simulink model "ComissionamentoMesa_simul"  (R2024a)
settings: Solver=FixedStepDiscrete  StartTime=0.0  StopTime=50  FixedStep=50e-3  RelTol=1e-3
undefined symbols (not defined in the file): flap_front_left_down, flap_front_left_up, flap_front_right_down, flap_front_right_up, flap_rear_left_down, flap_rear_left_up, flap_rear_right_down, flap_rear_right_up, tstep
libraries: speedgoatlib_IO60X_IO69X x1, tramontina_database_curtis_mesalib x1
settings Model: Creator=matlab.cut  LastModifiedBy=matlab.cut

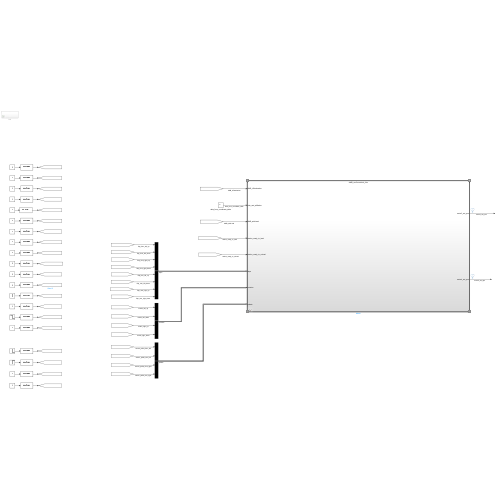
[thumbnail: Simulink's stored preview of the top-level diagram]
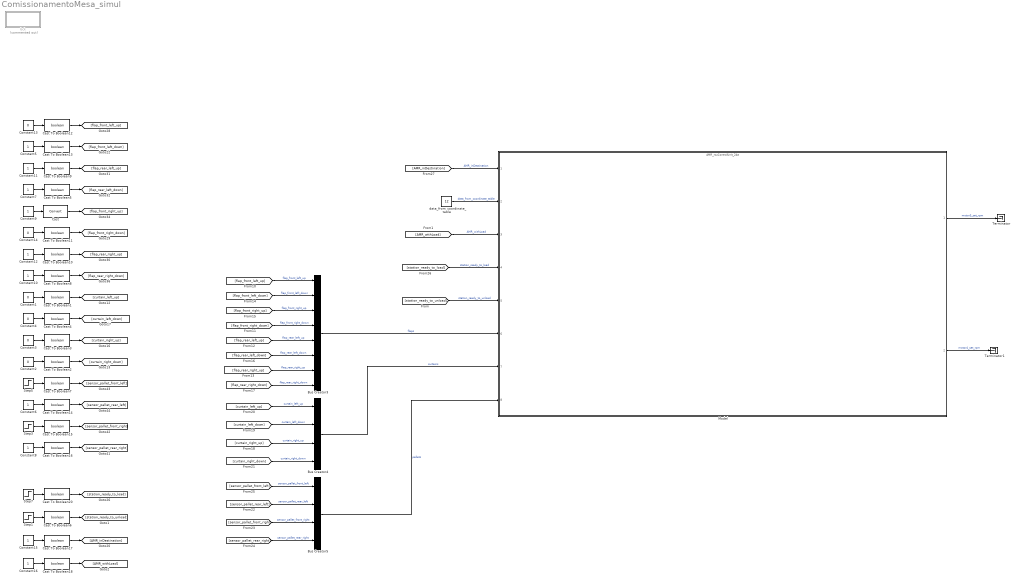
== system ComissionamentoMesa_simul ==
  Bus Creator3 : BusCreator  Inputs=flap_front_left_up,flap_front_left_down,flap_front_right_up,flap_front_right_down,flap_rear_left_up,flap_rear_left_down,flap_rear_right_up,flap_rear_right_down  OutDataTypeStr=Bus: IOs_flaps_bool
  Bus Creator4 : BusCreator  Inputs=4
  Bus Creator5 : BusCreator  Inputs=4
  Cast : DataTypeConversion  SaturateOnIntegerOverflow=off  RndMeth=Floor
  Cast To Boolean{1..18,20} (19 alike) : DataTypeConversion  OutDataTypeStr=boolean  SaturateOnIntegerOverflow=off  RndMeth=Floor
  Constant{1..4,13..14} (6 alike) : Constant  Value=0
  Constant{5..12,15..16} (10 alike) : Constant
  Model : ModelReference  ModelNameDialog=AMR_rcuControlUnit_24a.slx  SimulationMode=Normal  ModelReferenceVersion=1.13
  Step1 : Step  Time=40
  Step3 : Step  Time=35  Before=1  After=0  SampleTime=500e-3
  Step5 : Step  Time=35  Before=1  After=0  SampleTime=500e-3
  Step7 : Step  Time=30  Before=1  After=0
  Terminator : Terminator
  Terminator1 : Terminator
  bck : Subsystem  Commented=on
  data_from_coordinate_table : Constant  Value=12
  wires:
  Cast To Boolean7/1 -> [sensor_pallet_front_left]
  Step3/1 -> Cast To Boolean15/1
  Constant6/1 -> Cast To Boolean14/1
  Cast To Boolean15/1 -> [sensor_pallet_front_right]
  Cast To Boolean13/1 -> [flap_front_left_down]
  Constant5/1 -> Cast To Boolean13/1
  Constant13/1 -> Cast To Boolean12/1
  Constant10/1 -> Cast To Boolean8/1
  Cast To Boolean9/1 -> [flap_rear_left_up]
  Cast To Boolean11/1 -> [flap_front_right_down]
  Step5/1 -> Cast To Boolean7/1
  Cast To Boolean1/1 -> [curtain_left_up]
  Cast To Boolean14/1 -> [sensor_pallet_rear_left]
  Constant7/1 -> Cast To Boolean5/1
  Constant8/1 -> Cast To Boolean16/1
  Cast To Boolean10/1 -> [flap_rear_right_up]
  Cast To Boolean16/1 -> [sensor_pallet_rear_right]
  Constant11/1 -> Cast To Boolean9/1
  Constant14/1 -> Cast To Boolean11/1
  Constant2/1 -> Cast To Boolean2/1
  Cast To Boolean3/1 -> [curtain_right_up]
  Cast To Boolean4/1 -> [curtain_left_down]
  Constant3/1 -> Cast To Boolean3/1
  Cast To Boolean8/1 -> [flap_rear_right_down]
  Cast To Boolean2/1 -> [curtain_right_down]
  Constant1/1 -> Cast To Boolean1/1
  Cast To Boolean12/1 -> [flap_front_left_up]
  Cast To Boolean5/1 -> [flap_rear_left_down]
  Constant12/1 -> Cast To Boolean10/1
  Constant4/1 -> Cast To Boolean4/1
  [curtain_left_up] -> Bus Creator4/1  "curtain_left_up"
  [flap_front_left_down] -> Bus Creator3/2  "flap_front_left_down"
  [flap_rear_right_down] -> Bus Creator3/8  "flap_rear_right_down"
  [sensor_pallet_rear_right] -> Bus Creator5/4  "sensor_pallet_rear_right"
  [curtain_right_down] -> Bus Creator4/4  "curtain_right_down"
  [AMR_inDestination] -> Model/1  "AMR_inDestination"
  [flap_rear_right_up] -> Bus Creator3/7  "flap_rear_right_up"
  [flap_rear_left_down] -> Bus Creator3/6  "flap_rear_left_down"
  [sensor_pallet_front_right] -> Bus Creator5/3  "sensor_pallet_front_right"
  [flap_rear_left_up] -> Bus Creator3/5  "flap_rear_left_up"
  [flap_front_right_up] -> Bus Creator3/3  "flap_front_right_up"
  [flap_front_left_up] -> Bus Creator3/1  "flap_front_left_up"
  [sensor_pallet_rear_left] -> Bus Creator5/2  "sensor_pallet_rear_left"
  [sensor_pallet_front_left] -> Bus Creator5/1  "sensor_pallet_front_left"
  [curtain_right_up] -> Bus Creator4/3  "curtain_right_up"
  data_from_coordinate_table/1 -> Model/2  "data_from_coordinate_table"
  [flap_front_right_down] -> Bus Creator3/4  "flap_front_right_down"
  [curtain_left_down] -> Bus Creator4/2  "curtain_left_down"
  Constant15/1 -> Cast To Boolean17/1
  Cast To Boolean17/1 -> [AMR_inDestination]
  Cast To Boolean20/1 -> [station_ready_to_load]
  Step7/1 -> Cast To Boolean20/1
  Model/1 -> Terminator/1  "motor3_set_rpm"
  Model/2 -> Terminator1/1  "motor4_set_rpm"
  Cast/1 -> [flap_front_right_up]
  Constant9/1 -> Cast/1
  Cast To Boolean6/1 -> [station_ready_to_unload]
  Step1/1 -> Cast To Boolean6/1
  Cast To Boolean18/1 -> [AMR_withLoad]
  Constant16/1 -> Cast To Boolean18/1
  [AMR_withLoad] -> Model/3  "AMR_withLoad"
  [station_ready_to_load] -> Model/4  "station_ready_to_load"
  [station_ready_to_unload] -> Model/5  "station_ready_to_unload"
  Bus Creator3/1 -> Model/6  "flaps"
  Bus Creator4/1 -> Model/7  "curtains"
  Bus Creator5/1 -> Model/8  "pallets"

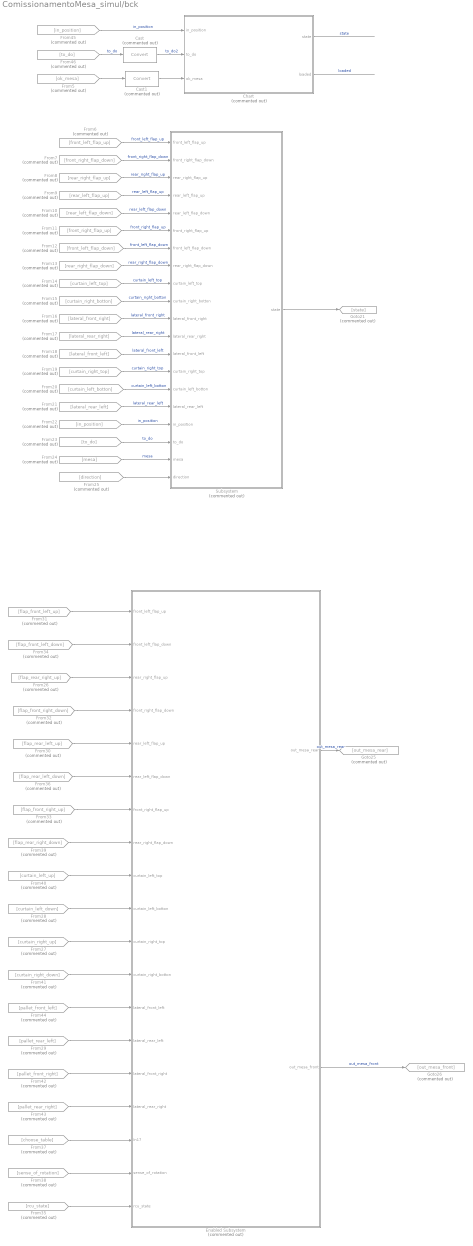
== system ComissionamentoMesa_simul/bck ==
  Cast : DataTypeConversion  Commented=on  SaturateOnIntegerOverflow=off  RndMeth=Floor
  Cast1 : DataTypeConversion  Commented=on  SaturateOnIntegerOverflow=off  RndMeth=Floor
  Chart : Stateflow chart  Commented=on  TreatAsAtomicUnit=on
  Enabled Subsystem : Subsystem  Commented=on  TreatAsAtomicUnit=on
  From10 : From  Commented=on  GotoTag=rear_left_flap_down
  From11 : From  Commented=on  GotoTag=front_right_flap_up
  From12 : From  Commented=on  GotoTag=front_left_flap_down
  From13 : From  Commented=on  GotoTag=rear_right_flap_down
  From14 : From  Commented=on  GotoTag=curtain_left_top
  From15 : From  Commented=on  GotoTag=curtain_right_botton
  From16 : From  Commented=on  GotoTag=lateral_front_right
  From17 : From  Commented=on  GotoTag=lateral_rear_right
  From18 : From  Commented=on  GotoTag=lateral_front_left
  From19 : From  Commented=on  GotoTag=curtain_right_top
  From20 : From  Commented=on  GotoTag=curtain_left_botton
  From21 : From  Commented=on  GotoTag=lateral_rear_left
  From22 : From  Commented=on  GotoTag=in_position
  From23 : From  Commented=on  GotoTag=to_do
  From24 : From  Commented=on  GotoTag=mesa
  From25 : From  Commented=on  GotoTag=direction
  From26 : From  Commented=on  GotoTag=flap_rear_right_up
  From27 : From  Commented=on  GotoTag=curtain_right_up
  From28 : From  Commented=on  GotoTag=curtain_left_down
  From29 : From  Commented=on  GotoTag=pallet_rear_left
  From30 : From  Commented=on  GotoTag=flap_rear_left_up
  From31 : From  Commented=on  GotoTag=flap_front_left_up
  From32 : From  Commented=on  GotoTag=flap_front_right_down
  From33 : From  Commented=on  GotoTag=flap_front_right_up
  From34 : From  Commented=on  GotoTag=flap_front_left_down
  From35 : From  Commented=on  GotoTag=rcu_state
  From36 : From  Commented=on  GotoTag=flap_rear_left_down
  From37 : From  Commented=on  GotoTag=choose_table
  From38 : From  Commented=on  GotoTag=sense_of_rotation
  From39 : From  Commented=on  GotoTag=flap_rear_right_down
  From40 : From  Commented=on  GotoTag=curtain_left_up
  From41 : From  Commented=on  GotoTag=curtain_right_down
  From42 : From  Commented=on  GotoTag=pallet_front_right
  From43 : From  Commented=on  GotoTag=pallet_rear_right
  From44 : From  Commented=on  GotoTag=pallet_front_left
  From45 : From  Commented=on  GotoTag=in_position
  From46 : From  Commented=on  GotoTag=to_do
  From5 : From  Commented=on  GotoTag=ok_mesa
  From6 : From  Commented=on  GotoTag=front_left_flap_up
  From7 : From  Commented=on  GotoTag=front_right_flap_down
  From8 : From  Commented=on  GotoTag=rear_right_flap_up
  From9 : From  Commented=on  GotoTag=rear_left_flap_up
  Goto21 : Goto  Commented=on  GotoTag=state
  Goto25 : Goto  Commented=on  GotoTag=out_mesa_rear
  Goto26 : Goto  Commented=on  GotoTag=out_mesa_front
  Subsystem : Subsystem  Commented=on
  wires:
  Chart/2(loaded) -> ?  "loaded"
  From31/1 -> Enabled Subsystem/1(front_left_flap_up)
  From27/1 -> Enabled Subsystem/11(curtain_right_top)
  From29/1 -> Enabled Subsystem/14(lateral_rear_left)
  From44/1 -> Enabled Subsystem/13(lateral_front_left)
  Enabled Subsystem/1(out_mesa_rear) -> Goto25/1  "out_mesa_rear"
  From30/1 -> Enabled Subsystem/5(rear_left_flap_up)
  From38/1 -> Enabled Subsystem/18(sense_of_rotation)
  From45/1 -> Chart/1(in_position)  "in_position"
  From6/1 -> Subsystem/1(front_left_flap_up)  "front_left_flap_up"
  Subsystem/1(state) -> Goto21/1
  From5/1 -> Cast1/1
  From43/1 -> Enabled Subsystem/16(lateral_rear_right)
  From32/1 -> Enabled Subsystem/4(front_right_flap_down)
  From13/1 -> Subsystem/8(rear_right_flap_down)  "rear_right_flap_down"
  From41/1 -> Enabled Subsystem/12(curtain_right_botton)
  From26/1 -> Enabled Subsystem/3(rear_right_flap_up)
  From34/1 -> Enabled Subsystem/2(front_left_flap_down)
  From20/1 -> Subsystem/15(curtain_left_botton)  "curtain_left_botton"
  From39/1 -> Enabled Subsystem/8(rear_right_flap_down)
  From37/1 -> Enabled Subsystem/17(In17)
  From24/1 -> Subsystem/19(mesa)  "mesa"
  From16/1 -> Subsystem/11(lateral_front_right)  "lateral_front_right"
  From22/1 -> Subsystem/17(in_position)  "in_position"
  From35/1 -> Enabled Subsystem/19(rcu_state)
  From42/1 -> Enabled Subsystem/15(lateral_front_right)
  From17/1 -> Subsystem/12(lateral_rear_right)  "lateral_rear_right"
  From21/1 -> Subsystem/16(lateral_rear_left)  "lateral_rear_left"
  From40/1 -> Enabled Subsystem/9(curtain_left_top)
  From14/1 -> Subsystem/9(curtain_left_top)  "curtain_left_top"
  Chart/1(state) -> ?  "state"
  From8/1 -> Subsystem/3(rear_right_flap_up)  "rear_right_flap_up"
  From18/1 -> Subsystem/13(lateral_front_left)  "lateral_front_left"
  From19/1 -> Subsystem/14(curtain_right_top)  "curtain_right_top"
  From10/1 -> Subsystem/5(rear_left_flap_down)  "rear_left_flap_down"
  From25/1 -> Subsystem/20(direction)
  From7/1 -> Subsystem/2(front_right_flap_down)  "front_right_flap_down"
  From46/1 -> Cast/1  "to_do"
  From9/1 -> Subsystem/4(rear_left_flap_up)  "rear_left_flap_up"
  Cast1/1 -> Chart/3(ok_mesa)
  From12/1 -> Subsystem/7(front_left_flap_down)  "front_left_flap_down"
  From28/1 -> Enabled Subsystem/10(curtain_left_botton)
  From11/1 -> Subsystem/6(front_right_flap_up)  "front_right_flap_up"
  Cast/1 -> Chart/2(to_do)  "to_do2"
  From15/1 -> Subsystem/10(curtain_right_botton)  "curtain_right_botton"
  From33/1 -> Enabled Subsystem/7(front_right_flap_up)
  From36/1 -> Enabled Subsystem/6(rear_left_flap_down)
  Enabled Subsystem/2(out_mesa_front) -> Goto26/1  "out_mesa_front"
  From23/1 -> Subsystem/18(to_do)  "to_do"

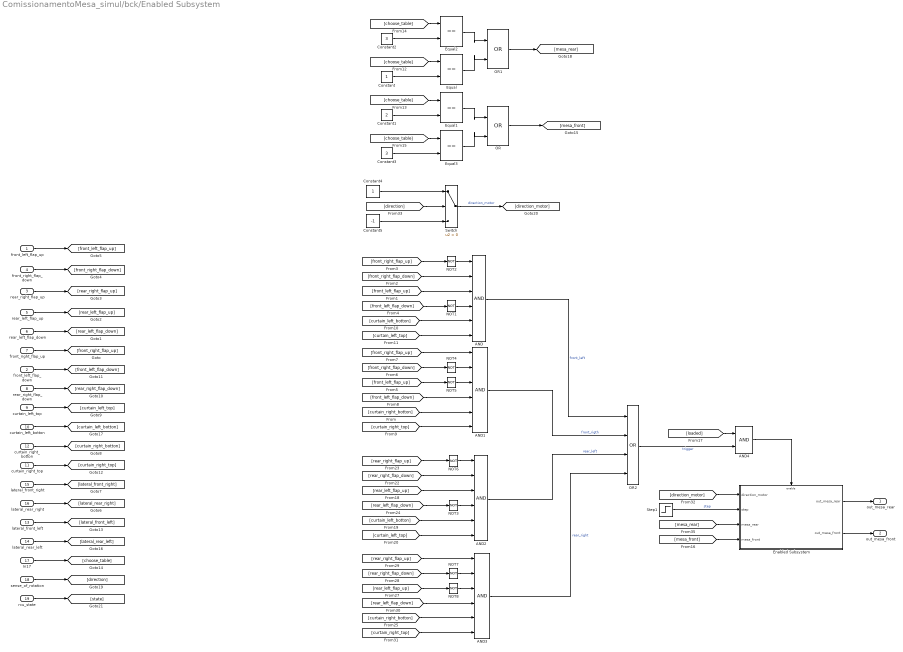
== system ComissionamentoMesa_simul/bck/Enabled Subsystem ==
  front_left_flap_up : Inport
  front_left_flap_down : Inport  Port=2
  rear_right_flap_up : Inport  Port=3
  front_right_flap_down : Inport  Port=4
  rear_left_flap_up : Inport  Port=5
  rear_left_flap_down : Inport  Port=6
  front_right_flap_up : Inport  Port=7
  rear_right_flap_down : Inport  Port=8
  curtain_left_top : Inport  Port=9
  curtain_left_botton : Inport  Port=10
  curtain_right_top : Inport  Port=11
  curtain_right_botton : Inport  Port=12
  lateral_front_left : Inport  Port=13
  lateral_rear_left : Inport  Port=14
  lateral_front_right : Inport  Port=15
  lateral_rear_right : Inport  Port=16
  In17 : Inport  Port=17
  sense_of_rotation : Inport  Port=18
  rcu_state : Inport  Port=19
  AND{,1..3} (4 alike) : Logic  Inputs=6  AllPortsSameDT=off  OutDataTypeStr=boolean
  AND4 : Logic  AllPortsSameDT=off  OutDataTypeStr=boolean
  Constant : Constant
  Constant1 : Constant  Value=2
  Constant2 : Constant  Value=3
  Constant3 : Constant  Value=3
  Constant4 : Constant
  Constant5 : Constant  Value=-1
  Enabled Subsystem : Subsystem  TreatAsAtomicUnit=on
  Equal{,1..3} (4 alike) : RelationalOperator  Operator===  OutDataTypeStr=boolean  RndMeth=Simplest  InputSameDT=off
  NOT{1..8} (8 alike) : Logic  Operator=NOT  IconShape=distinctive  AllPortsSameDT=off  OutDataTypeStr=boolean
  OR : Logic  Operator=OR  IconShape=distinctive  AllPortsSameDT=off  OutDataTypeStr=boolean
  OR1 : Logic  Operator=OR  IconShape=distinctive  AllPortsSameDT=off  OutDataTypeStr=boolean
  OR2 : Logic  Operator=OR  Inputs=4  AllPortsSameDT=off  OutDataTypeStr=boolean
  Step1 : Step  Time=20
  Switch : Switch  Criteria=u2 > Threshold  SaturateOnIntegerOverflow=off  InputSameDT=off
  out_mesa_rear : Outport
  out_mesa_front : Outport  Port=2
  wires:
  NOT2/1 -> AND/1
  [front_left_flap_up] -> AND/3
  NOT1/1 -> AND/4
  [front_left_flap_down] -> NOT1/1
  [front_right_flap_down] -> AND/2
  [front_right_flap_up] -> NOT2/1
  front_right_flap_down/1 -> [front_right_flap_down]
  front_left_flap_up/1 -> [front_left_flap_up]
  rear_right_flap_up/1 -> [rear_right_flap_up]
  rear_left_flap_up/1 -> [rear_left_flap_up]
  rear_left_flap_down/1 -> [rear_left_flap_down]
  front_right_flap_up/1 -> [front_right_flap_up]
  front_left_flap_down/1 -> [front_left_flap_down]
  rear_right_flap_down/1 -> [rear_right_flap_down]
  curtain_left_top/1 -> [curtain_left_top]
  curtain_right_botton/1 -> [curtain_right_botton]
  lateral_front_right/1 -> [lateral_front_right]
  lateral_rear_right/1 -> [lateral_rear_right]
  lateral_front_left/1 -> [lateral_front_left]
  curtain_right_top/1 -> [curtain_right_top]
  curtain_left_botton/1 -> [curtain_left_botton]
  lateral_rear_left/1 -> [lateral_rear_left]
  [front_right_flap_down] -> NOT4/1
  [front_left_flap_down] -> AND1/4
  [front_left_flap_up] -> NOT5/1
  [front_right_flap_up] -> AND1/1
  NOT5/1 -> AND1/3
  NOT4/1 -> AND1/2
  [curtain_right_botton] -> AND1/5
  [curtain_right_top] -> AND1/6
  [curtain_left_botton] -> AND/5
  [curtain_left_top] -> AND/6
  In17/1 -> [choose_table]
  [choose_table] -> Equal/1
  Constant/1 -> Equal/2
  [choose_table] -> Equal1/1
  Constant1/1 -> Equal1/2
  [choose_table] -> Equal2/1
  Constant2/1 -> Equal2/2
  Constant3/1 -> Equal3/2
  [choose_table] -> Equal3/1
  Equal1/1 -> OR/1
  Equal3/1 -> OR/2
  Equal/1 -> OR1/2
  Equal2/1 -> OR1/1
  OR/1 -> [mesa_front]
  OR1/1 -> [mesa_rear]
  [curtain_left_top] -> AND2/6
  [curtain_left_botton] -> AND2/5
  [rear_right_flap_up] -> NOT6/1
  [rear_right_flap_down] -> AND2/2
  [rear_left_flap_down] -> NOT3/1
  NOT3/1 -> AND2/4
  [rear_left_flap_up] -> AND2/3
  NOT6/1 -> AND2/1
  [curtain_right_top] -> AND3/6
  [curtain_right_botton] -> AND3/5
  NOT7/1 -> AND3/2
  NOT8/1 -> AND3/3
  [rear_right_flap_up] -> AND3/1
  [rear_left_flap_up] -> NOT8/1
  [rear_left_flap_down] -> AND3/4
  [rear_right_flap_down] -> NOT7/1
  sense_of_rotation/1 -> [direction]
  [direction] -> Switch/2
  Constant4/1 -> Switch/1
  Constant5/1 -> Switch/3
  Switch/1 -> [direction_motor]  "direction_motor"
  AND/1 -> OR2/1  "front_left"
  AND1/1 -> OR2/2  "front_rigth"
  AND2/1 -> OR2/3  "rear_left"
  AND3/1 -> OR2/4  "rear_right"
  OR2/1 -> AND4/2  "trigger"
  [direction_motor] -> Enabled Subsystem/1(direction_motor)
  Step1/1 -> Enabled Subsystem/2(step)  "step"
  [mesa_rear] -> Enabled Subsystem/3(mesa_rear)
  [mesa_front] -> Enabled Subsystem/4(mesa_front)
  Enabled Subsystem/1(out_mesa_rear) -> out_mesa_rear/1
  Enabled Subsystem/2(out_mesa_front) -> out_mesa_front/1
  rcu_state/1 -> [state]
  [loaded] -> AND4/1
  AND4/1 -> Enabled Subsystem/Enable

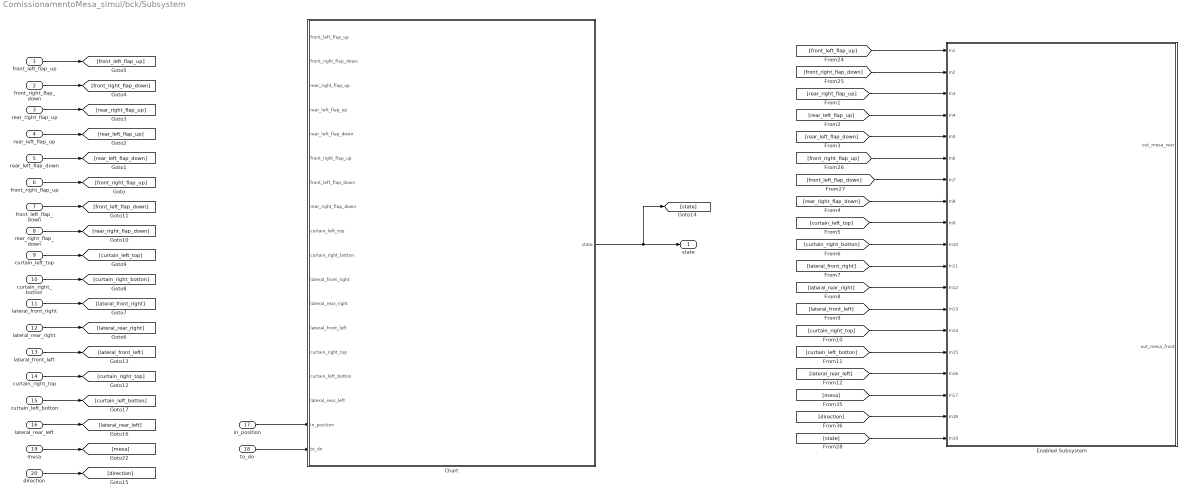
== system ComissionamentoMesa_simul/bck/Subsystem ==
  front_left_flap_up : Inport
  front_right_flap_down : Inport  Port=2
  rear_right_flap_up : Inport  Port=3
  rear_left_flap_up : Inport  Port=4
  rear_left_flap_down : Inport  Port=5
  front_right_flap_up : Inport  Port=6
  front_left_flap_down : Inport  Port=7
  rear_right_flap_down : Inport  Port=8
  curtain_left_top : Inport  Port=9
  curtain_right_botton : Inport  Port=10
  lateral_front_right : Inport  Port=11
  lateral_rear_right : Inport  Port=12
  lateral_front_left : Inport  Port=13
  curtain_right_top : Inport  Port=14
  curtain_left_botton : Inport  Port=15
  lateral_rear_left : Inport  Port=16
  in_position : Inport  Port=17
  to_do : Inport  Port=18
  mesa : Inport  Port=19
  direction : Inport  Port=20
  Chart : Stateflow chart  TreatAsAtomicUnit=on
  Enabled Subsystem : Subsystem  TreatAsAtomicUnit=on
  state : Outport
  wires:
  Chart/1(state) -> [state], state/1
  [state] -> Enabled Subsystem/19(In19)
  [front_right_flap_down] -> Enabled Subsystem/2(In2)
  [front_left_flap_up] -> Enabled Subsystem/1(In1)
  front_right_flap_up/1 -> [front_right_flap_up]
  lateral_rear_right/1 -> [lateral_rear_right]
  lateral_front_right/1 -> [lateral_front_right]
  curtain_right_botton/1 -> [curtain_right_botton]
  curtain_left_top/1 -> [curtain_left_top]
  rear_right_flap_down/1 -> [rear_right_flap_down]
  front_left_flap_down/1 -> [front_left_flap_down]
  rear_left_flap_down/1 -> [rear_left_flap_down]
  rear_left_flap_up/1 -> [rear_left_flap_up]
  rear_right_flap_up/1 -> [rear_right_flap_up]
  front_right_flap_down/1 -> [front_right_flap_down]
  front_left_flap_up/1 -> [front_left_flap_up]
  curtain_left_botton/1 -> [curtain_left_botton]
  in_position/1 -> Chart/17(in_position)
  to_do/1 -> Chart/18(to_do)
  lateral_rear_left/1 -> [lateral_rear_left]
  curtain_right_top/1 -> [curtain_right_top]
  lateral_front_left/1 -> [lateral_front_left]
  [rear_right_flap_down] -> Enabled Subsystem/8(In8)
  [curtain_left_top] -> Enabled Subsystem/9(In9)
  [curtain_right_botton] -> Enabled Subsystem/10(In10)
  [lateral_front_right] -> Enabled Subsystem/11(In11)
  [lateral_rear_right] -> Enabled Subsystem/12(In12)
  [lateral_front_left] -> Enabled Subsystem/13(In13)
  [curtain_right_top] -> Enabled Subsystem/14(In14)
  [curtain_left_botton] -> Enabled Subsystem/15(In15)
  [lateral_rear_left] -> Enabled Subsystem/16(In16)
  [front_left_flap_down] -> Enabled Subsystem/7(In7)
  [rear_right_flap_up] -> Enabled Subsystem/3(In3)
  [front_right_flap_up] -> Enabled Subsystem/6(In6)
  [rear_left_flap_up] -> Enabled Subsystem/4(In4)
  [rear_left_flap_down] -> Enabled Subsystem/5(In5)
  mesa/1 -> [mesa]
  [mesa] -> Enabled Subsystem/17(In17)
  direction/1 -> [direction]
  [direction] -> Enabled Subsystem/18(In18)

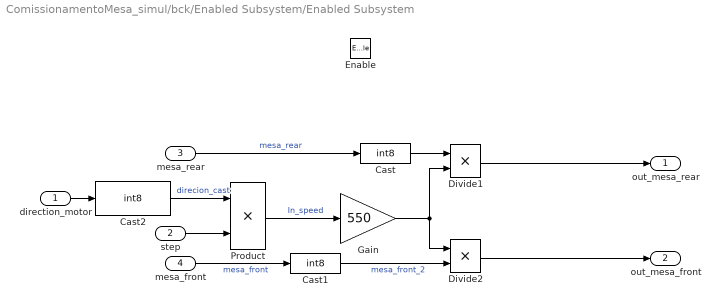
== system ComissionamentoMesa_simul/bck/Enabled Subsystem/Enabled Subsystem ==
  direction_motor : Inport
  step : Inport  Port=2
  mesa_rear : Inport  Port=3
  mesa_front : Inport  Port=4
  Enable : EnablePort
  Cast : DataTypeConversion  OutDataTypeStr=int8  SaturateOnIntegerOverflow=off  RndMeth=Floor
  Cast1 : DataTypeConversion  OutDataTypeStr=int8  SaturateOnIntegerOverflow=off  RndMeth=Floor
  Cast2 : DataTypeConversion  OutDataTypeStr=int8  SaturateOnIntegerOverflow=off  RndMeth=Floor
  Divide1 : Product  Inputs=**
  Divide2 : Product  Inputs=**
  Gain : Gain  Gain=550
  Product : Product
  out_mesa_rear : Outport  OutputWhenDisabled=reset  InitialOutput=[0]
  out_mesa_front : Outport  Port=2  OutputWhenDisabled=reset  InitialOutput=[0]
  wires:
  Product/1 -> Gain/1  "In_speed"
  direction_motor/1 -> Cast2/1
  step/1 -> Product/2
  mesa_rear/1 -> Cast/1  "mesa_rear"
  Gain/1 -> Divide1/2, Divide2/1
  Divide1/1 -> out_mesa_rear/1
  mesa_front/1 -> Cast1/1  "mesa_front"
  Divide2/1 -> out_mesa_front/1
  Cast/1 -> Divide1/1
  Cast1/1 -> Divide2/2  "mesa_front_2"
  Cast2/1 -> Product/1  "direcion_cast"

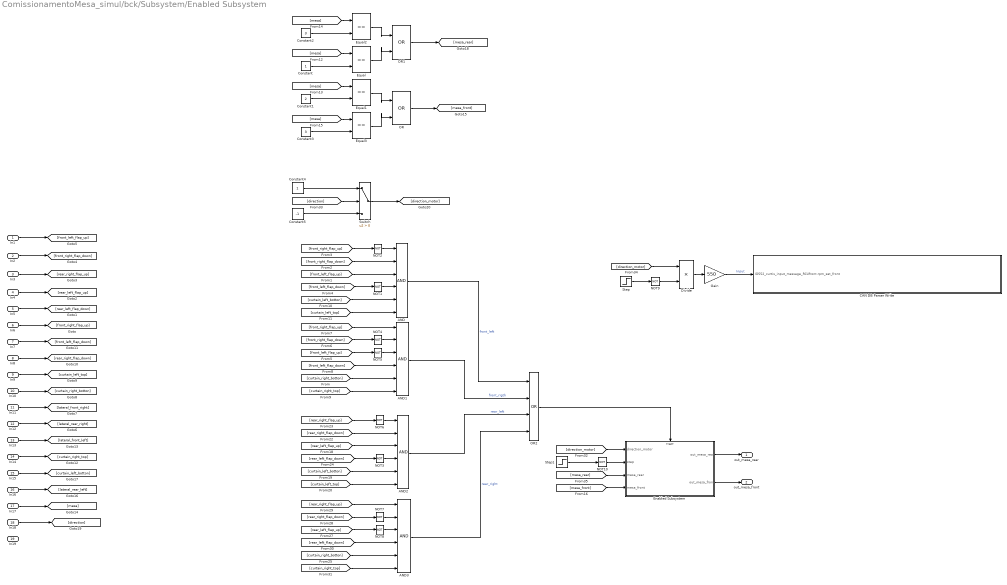
== system ComissionamentoMesa_simul/bck/Subsystem/Enabled Subsystem ==
  In1 : Inport
  In2 : Inport  Port=2
  In3 : Inport  Port=3
  In4 : Inport  Port=4
  In5 : Inport  Port=5
  In6 : Inport  Port=6
  In7 : Inport  Port=7
  In8 : Inport  Port=8
  In9 : Inport  Port=9
  In10 : Inport  Port=10
  In11 : Inport  Port=11
  In12 : Inport  Port=12
  In13 : Inport  Port=13
  In14 : Inport  Port=14
  In15 : Inport  Port=15
  In16 : Inport  Port=16
  In17 : Inport  Port=17
  In18 : Inport  Port=18
  In19 : Inport  Port=19
  AND{,1..3} (4 alike) : Logic  Inputs=6  AllPortsSameDT=off  OutDataTypeStr=boolean
  "CAN DB Parser Write " : Subsystem
      settings: OpenFcn=sg_can.OpenFcnWrite;
      mask Help: eval('sg.utils.help.show(''io_main/refentry_ref_can_ofa_parsing_write'');')
      mask Display: disp('Speedgoat\nIO691\nCAN DB Parser Write\nModule ID: IO691 - Module ID 1\nChannel:  1\ntramontina_database_curtis_mesa.dbc ');
  Constant : Constant
  Constant1 : Constant  Value=2
  Constant2 : Constant  Value=3
  Constant3 : Constant  Value=3
  Constant4 : Constant
  Constant5 : Constant  Value=-1
  Divide : Product  Inputs=**
  Enabled Subsystem : Subsystem  TreatAsAtomicUnit=on
  Equal{,1..3} (4 alike) : RelationalOperator  Operator===  OutDataTypeStr=boolean  RndMeth=Simplest  InputSameDT=off
  Gain : Gain  Gain=550
  NOT{1..10} (10 alike) : Logic  Operator=NOT  IconShape=distinctive  AllPortsSameDT=off  OutDataTypeStr=boolean
  OR : Logic  Operator=OR  IconShape=distinctive  AllPortsSameDT=off  OutDataTypeStr=boolean
  OR1 : Logic  Operator=OR  IconShape=distinctive  AllPortsSameDT=off  OutDataTypeStr=boolean
  OR2 : Logic  Operator=OR  Inputs=4  AllPortsSameDT=off  OutDataTypeStr=boolean
  Step : Step  Time=30  SampleTime=tstep
  Step1 : Step  Time=30  SampleTime=tstep
  Switch : Switch  Criteria=u2 > Threshold  SaturateOnIntegerOverflow=off  InputSameDT=off
  out_mesa_rear : Outport
  out_mesa_front : Outport  Port=2
  wires:
  NOT2/1 -> AND/1
  [front_left_flap_up] -> AND/3
  NOT1/1 -> AND/4
  [front_left_flap_down] -> NOT1/1
  [front_right_flap_down] -> AND/2
  [front_right_flap_up] -> NOT2/1
  In2/1 -> [front_right_flap_down]
  In1/1 -> [front_left_flap_up]
  In3/1 -> [rear_right_flap_up]
  In4/1 -> [rear_left_flap_up]
  In5/1 -> [rear_left_flap_down]
  In6/1 -> [front_right_flap_up]
  In7/1 -> [front_left_flap_down]
  In8/1 -> [rear_right_flap_down]
  In9/1 -> [curtain_left_top]
  In10/1 -> [curtain_right_botton]
  In11/1 -> [lateral_front_right]
  In12/1 -> [lateral_rear_right]
  In13/1 -> [lateral_front_left]
  In14/1 -> [curtain_right_top]
  In15/1 -> [curtain_left_botton]
  In16/1 -> [lateral_rear_left]
  [front_right_flap_down] -> NOT4/1
  [front_left_flap_down] -> AND1/4
  [front_left_flap_up] -> NOT5/1
  [front_right_flap_up] -> AND1/1
  NOT5/1 -> AND1/3
  NOT4/1 -> AND1/2
  [curtain_right_botton] -> AND1/5
  [curtain_right_top] -> AND1/6
  [curtain_left_botton] -> AND/5
  [curtain_left_top] -> AND/6
  In17/1 -> [mesa]
  [mesa] -> Equal/1
  Constant/1 -> Equal/2
  [mesa] -> Equal1/1
  Constant1/1 -> Equal1/2
  [mesa] -> Equal2/1
  Constant2/1 -> Equal2/2
  Constant3/1 -> Equal3/2
  [mesa] -> Equal3/1
  Equal1/1 -> OR/1
  Equal3/1 -> OR/2
  Equal/1 -> OR1/2
  Equal2/1 -> OR1/1
  OR/1 -> [mesa_front]
  OR1/1 -> [mesa_rear]
  [curtain_left_top] -> AND2/6
  [curtain_left_botton] -> AND2/5
  [rear_right_flap_up] -> NOT6/1
  [rear_right_flap_down] -> AND2/2
  [rear_left_flap_down] -> NOT3/1
  NOT3/1 -> AND2/4
  [rear_left_flap_up] -> AND2/3
  NOT6/1 -> AND2/1
  [curtain_right_top] -> AND3/6
  [curtain_right_botton] -> AND3/5
  NOT7/1 -> AND3/2
  NOT8/1 -> AND3/3
  [rear_right_flap_up] -> AND3/1
  [rear_left_flap_up] -> NOT8/1
  [rear_left_flap_down] -> AND3/4
  [rear_right_flap_down] -> NOT7/1
  Gain/1 -> "CAN DB Parser Write "/1(ID552_curtis_input_message_RCUfront.rpm_set_front)  "Input"
  In18/1 -> [direction]
  [direction] -> Switch/2
  Constant4/1 -> Switch/1
  Constant5/1 -> Switch/3
  Switch/1 -> [direction_motor]
  [direction_motor] -> Divide/1
  Divide/1 -> Gain/1
  Step/1 -> NOT9/1
  NOT9/1 -> Divide/2
  AND/1 -> OR2/1  "front_left"
  AND1/1 -> OR2/2  "front_rigth"
  AND2/1 -> OR2/3  "rear_left"
  AND3/1 -> OR2/4  "rear_right"
  OR2/1 -> Enabled Subsystem/Trigger
  [direction_motor] -> Enabled Subsystem/1(direction_motor)
  Step1/1 -> NOT10/1
  NOT10/1 -> Enabled Subsystem/2(step)
  [mesa_rear] -> Enabled Subsystem/3(mesa_rear)
  [mesa_front] -> Enabled Subsystem/4(mesa_front)
  Enabled Subsystem/1(out_mesa_rear) -> out_mesa_rear/1
  Enabled Subsystem/2(out_mesa_front) -> out_mesa_front/1

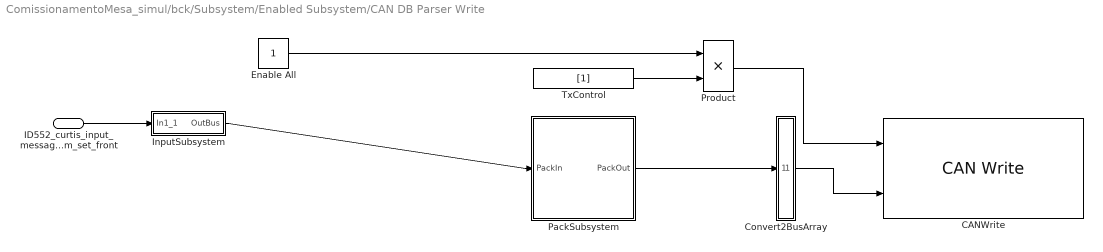
== system ComissionamentoMesa_simul/bck/Subsystem/Enabled Subsystem/CAN DB Parser Write  ==
  ID552_curtis_input_message_RCUfront.rpm_set_front : Inport
  CANWrite : speedgoatlib_IO60X_IO69X/CAN/CAN Write   moduleType=IO691  id=1  channel=1  canType=CAN (HS)  messageType=CAN (HS)  useBusIn=on  numOfMsg=1  enableInput=on  enableStatusPort=off  ts=-1  initValues=[691 1 -1 0 1 1 0 1 1 1]
  Convert2BusArray : Subsystem
  Enable All : Constant  OutDataTypeStr=boolean
  InputSubsystem : Subsystem
  PackSubsystem : Subsystem
  Product : Product  OutDataTypeStr=uint32
  TxControl : Constant  Value=[1]  OutDataTypeStr=uint32
  wires:
  PackSubsystem/1(PackOut) -> Convert2BusArray/1(InBus)
  Convert2BusArray/1(BusArrayOut) -> CANWrite/2
  Product/1 -> CANWrite/1
  TxControl/1 -> Product/2
  Enable All/1 -> Product/1
  ID552_curtis_input_message_RCUfront.rpm_set_front/1 -> InputSubsystem/1(In1_1)
  InputSubsystem/1(OutBus) -> PackSubsystem/1(PackIn)

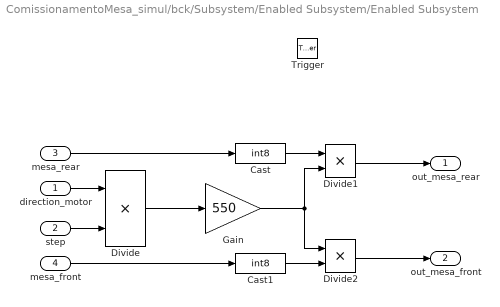
== system ComissionamentoMesa_simul/bck/Subsystem/Enabled Subsystem/Enabled Subsystem ==
  direction_motor : Inport
  step : Inport  Port=2
  mesa_rear : Inport  Port=3
  mesa_front : Inport  Port=4
  Trigger : TriggerPort  VariantControl=(inherit)  PortDimensions=1
  Cast : DataTypeConversion  OutDataTypeStr=int8  SaturateOnIntegerOverflow=off  RndMeth=Floor
  Cast1 : DataTypeConversion  OutDataTypeStr=int8  SaturateOnIntegerOverflow=off  RndMeth=Floor
  Divide : Product  Inputs=**
  Divide1 : Product  Inputs=**
  Divide2 : Product  Inputs=**
  Gain : Gain  Gain=550
  out_mesa_rear : Outport
  out_mesa_front : Outport  Port=2
  wires:
  Divide/1 -> Gain/1
  direction_motor/1 -> Divide/1
  step/1 -> Divide/2
  mesa_rear/1 -> Cast/1
  Gain/1 -> Divide1/2, Divide2/1
  Divide1/1 -> out_mesa_rear/1
  mesa_front/1 -> Cast1/1
  Divide2/1 -> out_mesa_front/1
  Cast/1 -> Divide1/1
  Cast1/1 -> Divide2/2

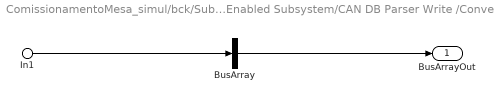
== system ComissionamentoMesa_simul/bck/Subsystem/Enabled Subsystem/CAN DB Parser Write /Convert2BusArray ==
  In1 : Inport  PortName=InBus  Element=ID552_curtis_input_message_RCUfront
  BusArray : Concatenate  NumInputs=1
  BusArrayOut : Outport
  wires:
  In1/1 -> BusArray/1
  BusArray/1 -> BusArrayOut/1

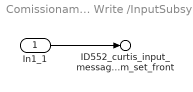
== system ComissionamentoMesa_simul/bck/Subsystem/Enabled Subsystem/CAN DB Parser Write /InputSubsystem ==
  In1_1 : Inport
  ID552_curtis_input_message_RCUfront.rpm_set_front : Outport  PortName=OutBus  Element=ID552_curtis_input_message_RCUfront.rpm_set_front
  wires:
  In1_1/1 -> ID552_curtis_input_message_RCUfront.rpm_set_front/1

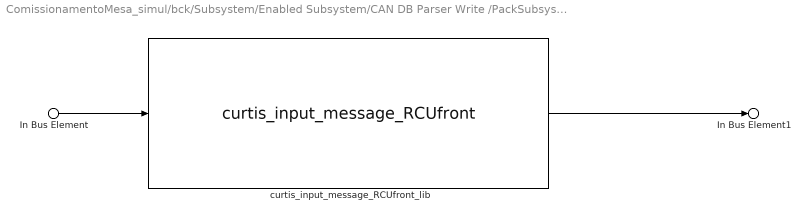
== system ComissionamentoMesa_simul/bck/Subsystem/Enabled Subsystem/CAN DB Parser Write /PackSubsystem ==
  In Bus Element : Inport  PortName=PackIn  Element=ID552_curtis_input_message_RCUfront
  curtis_input_message_RCUfront_lib : tramontina_database_curtis_mesalib/CAN pack/curtis_input_message_RCUfront  SystemSampleTime=-1  VariantActivationTime=update diagram  AllowFlexibleInterface=on  Latency=0  AutoFrameSizeCalculation=off
  In Bus Element1 : Outport  PortName=PackOut  Element=ID552_curtis_input_message_RCUfront
  wires:
  In Bus Element/1 -> curtis_input_message_RCUfront_lib/1
  curtis_input_message_RCUfront_lib/1 -> In Bus Element1/1

== stateflow chart ComissionamentoMesa_simul/bck/Subsystem/Chart ==
  state standby
    entry:
    state = 0;
    settings: description=This state models the modes of a window sensor and implements logic to respond when that sensor is producing a signal.
  state waiting [commented out]
    state=0;
  state Loading
    entry:
    state=1;
    exit:
    loaded=1;
  state Unloading
    entry:
    state=2;
    exit:
    loaded=0;
  state Idle [commented out]
    state=0;
  (default) -> standby
  (default) -> (junction 50) [commented out]
  standby -> (junction 58) [order 2]
  (junction 75) -> standby
  (junction 74) -> (junction 75)
  (junction 58) -> Unloading : [to_do==2|loaded==1|in_position==TRUE]
  standby -> Loading [order 1] : [to_do==1|loaded==0|in_position==TRUE]
  (junction 46) -> (junction 50) [commented out]
  (junction 50) -> waiting [commented out]
  Idle -> (junction 46) [commented out] : [loaded==-1]
  waiting -> Idle [commented out] : [in_position==TRUE]
  Unloading -> (junction 73) : [SensorOff]
  Loading -> (junction 81)
  (junction 81) -> (junction 74)
  (junction 73) -> (junction 81)
  data: front_left_flap_up input; front_right_flap_down input; rear_right_flap_up input; rear_left_flap_up input; rear_left_flap_down input; front_right_flap_up input; front_left_flap_down input; rear_right_flap_down input; curtain_left_top input; curtain_right_botton input; lateral_front_right input; lateral_rear_right input; lateral_front_left input; curtain_right_top input; curtain_left_botton input; lateral_rear_left input; in_position input; to_do input; state output; loaded local

== stateflow chart ComissionamentoMesa_simul/bck/Chart ==
  state %&&(lateral_front_left==1|lateral_front_right==1) [group] [commented out]
  state standby
    entry:
    state = 0;
    settings: description=This state models the modes of a window sensor and implements logic to respond when that sensor is producing a signal.
  state waiting [commented out]
    state=0;
  state Loading
    entry:
    state=1;
    exit:
    loaded=TRUE;
  state Unloading
    entry:
    state=2;
    exit:
    loaded=FALSE;
  state Idle [commented out]
    state=0;
  (default) -> standby : {loaded=0}
  (default) -> (junction 50) [commented out]
  standby -> (junction 58) [order 2]
  (junction 75) -> standby
  (junction 74) -> (junction 75)
  (junction 58) -> Unloading : [to_do==0 && loaded==1 && in_position==1]
  standby -> Loading [order 1] : [to_do==1 && loaded==0 && in_position==1]
  (junction 46) -> (junction 50) [commented out]
  (junction 50) -> waiting [commented out]
  Idle -> (junction 46) [commented out] : [loaded==-1]
  waiting -> Idle [commented out] : [in_position==TRUE]
  Unloading -> (junction 73) : [ok_mesa==TRUE]
  Loading -> (junction 81) : [ok_mesa==TRUE]
  (junction 81) -> (junction 74)
  (junction 73) -> (junction 81)
  data: in_position input; to_do input; state output; ok_mesa input; loaded output
